simulink model "FEEDBACK_LINEARIZATION"  (R2023b)
settings: Solver=VariableStepAuto  StartTime=0.0  StopTime=70  MaxStep=0.01  RelTol=1e-3
undefined symbols (not defined in the file): A_ego, B_ego, f_r, g, L, N, theta
libraries: sim3dautolib x2, drivingscenarioandsensors x2, mpclib x1, sim3dlib x1
settings Model: Creator=monis  LastModifiedBy=monis

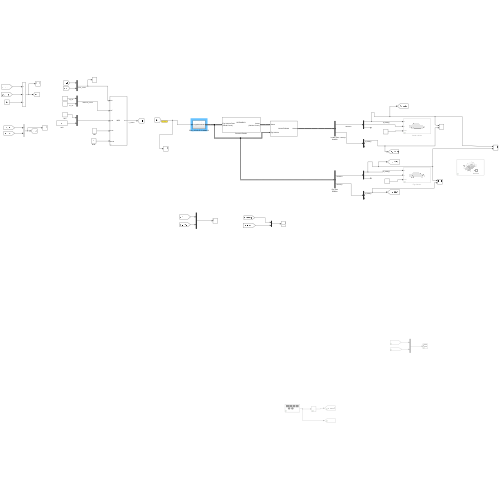
[thumbnail: Simulink's stored preview of the top-level diagram]
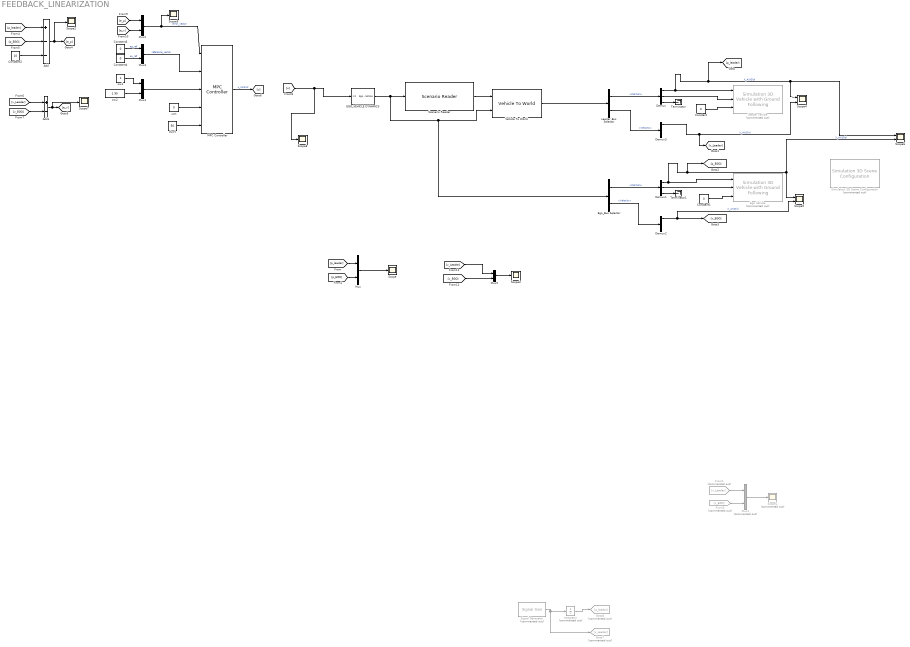
== system FEEDBACK_LINEARIZATION ==
  Add : Sum  Inputs=+--
  Add1 : Sum  Inputs=+-
  Constant{,1,3..4} (4 alike) : Constant  Value=0
  Constant2 : Constant  Value=10
  Demux{,1..3} (4 alike) : Demux  Outputs=3
  EGO_VEHICLE DYNAMICS : Subsystem
  Ego Vehicle : sim3dautolib/Simulation 3D Vehicle with Ground Following  Priority=-1  Commented=on  PassVehMesh=Muscle car  MeshPath=/MathWorksAutomotiveContent/Vehicles/Muscle/Meshes/SK_MuscleCar.SK_MuscleCar  TrackWidth=1.9  WheelBase=3  WheelRadius=0.35  VehColor=Orange  InitialPos=[0, 0, 0]  InitialRot=[0, 0, 0]  ActorName=EgoVehicle  SampleTime=-1  ActorType=SimulinkVehicle  ID=C  aMode=3  ActorTag=EgoVehicle  CoordinateScheme=ISO  VehLightsControl=off  HeadlightColor=[ 1, 1, 1 ]  HighBeamIntensity=100000  LowBeamIntensity=60000  HighBeamConeAngle=70  LowBeamConeAngle=70  LeftHeadlightOrientation=[ 0, 0 ]  RightHeadlightOrientation=[ 0, 0 ]  BrakelightIntensity=500  ReverselightIntensity=500  SignallightIntensity=500  SignallightPeriod=1  SignalPulseWidth=50  TransformOutportEnabled=off
      settings: LibrarySourceBlock=drivingsim3d/Simulation 3D Vehicle with Ground Following
  Ego_Bus Selector : BusSelector  OutputSignals=Position,Velocity
  From1 : From  Commented=on  GotoTag=v_Leader
  From3 : From  Commented=on  GotoTag=v_EGO
  Goto7 : Goto  Commented=on  GotoTag=v_Leader
  Goto8 : Goto  Commented=on  GotoTag=p_leader
  Integrator : Integrator  Commented=on  UpperSaturationLimit=+2500  LowerSaturationLimit=-2500
  Leader vehicle : sim3dautolib/Simulation 3D Vehicle with Ground Following  Priority=-1  Commented=on  PassVehMesh=Muscle car  MeshPath=/MathWorksAutomotiveContent/Vehicles/Muscle/Meshes/SK_MuscleCar.SK_MuscleCar  TrackWidth=1.9  WheelBase=3  WheelRadius=0.35  VehColor=Silver  InitialPos=[0, 0, 0]  InitialRot=[0, 0, 0]  ActorName=LeaderVehicle  SampleTime=-1  ActorType=SimulinkVehicle  ID=C  aMode=3  ActorTag=LeaderVehicle  CoordinateScheme=ISO  VehLightsControl=off  HeadlightColor=[ 1, 1, 1 ]  HighBeamIntensity=100000  LowBeamIntensity=60000  HighBeamConeAngle=70  LowBeamConeAngle=70  LeftHeadlightOrientation=[ 0, 0 ]  RightHeadlightOrientation=[ 0, 0 ]  BrakelightIntensity=500  ReverselightIntensity=500  SignallightIntensity=500  SignallightPeriod=1  SignalPulseWidth=50  TransformOutportEnabled=off
      settings: LibrarySourceBlock=drivingsim3d/Simulation 3D Vehicle with Ground Following
  Leader_Bus Selector : BusSelector  OutputSignals=Actors.Position,Actors.Velocity
  MPC Controller : mpclib/MPC Controller  SCDEnableBlockLinearizationSpecification=on  mpcobj=mpc2  is_multiple=0  enable_value=0  return_u0=off  updateMPCinCallerWorkspace=on  md_inport=off  mv_inport=off  uref_inport=off  return_cost=off  return_mvseq=off  return_qpstatus=off  return_xseq=off  return_state=off  return_ovseq=off  state_inport=off  umin_inport=off  umax_inport=off  ymin_inport=off  ymax_inport=off  cc_inport=off  ywt_inport=on  uwt_inport=on  duwt_inport=on  rhoeps_inport=off  pm_inport=off  MaximumP=10  HorizonChoice=FixedHorizon  n_ts=0.01  n_p=100  n_mv=1  n_md=0  n_ud=0  n_mo=2  n_uo=0  BlockDataType=double  SampleTimeInherited=off  switch_inport=off
  Mux{,2..5} (5 alike) : Mux  Inputs=2
  Mux1 : Mux  Commented=on  Inputs=2
  Scenario Reader : drivingscenarioandsensors/Scenario Reader  ScenarioSource=From file  ScenarioFileName=C:\Users\monis\Downloads\UNINA LEC\FINAL CONTROL SYS PROJECT 2023\SCENARIO1.mat  ScenarioVariableName=scenario  OutputCoordinateSystem=Vehicle coordinates  EgoVehicleSource=Input port  EgoVehicleActorID=1  OrientVehiclesOnRoad=off  OutputEgoVehiclePose=off  OutputEgoVehicleState=off  SampleTime=0.1  LaneBoundaryOutput=None  LaneBoundaryDistance=0:0.5:9.5  LaneBoundaryLocation=Center of lane markings  BusNameSource=Auto  BusName=BusActors  BusNumActorsSource=Scenario  BusNumActors=100  BusName2Source=Auto  BusName2=BusLaneBoundaries  BusNumLaneBoundariesSource=Scenario  BusNumLaneBoundaries=10  BusName3Source=Auto  BusName3=BusEgoActor  BusName4Source=Auto  BusName4=BusEgoState  ShowCoordinateLabels=on  SimulateUsing=Interpreted execution
  Scope{,2..3,7..9} (6 alike) : Scope
  Scope1 : Scope  Commented=on
  Scope4 : Scope  NumInputPorts=2
  Scope5 : Scope  NumInputPorts=2
  Scope6 : Scope  NumInputPorts=2
  Signal Generator : SignalGenerator  Commented=on  WaveForm=random  Units=rad/sec
  Simulation 3D Scene Configuration : sim3dlib/Simulation 3D Scene Configuration  Priority=0  Commented=on  ProjectFormat=Default Scenes  SceneDesc=Straight road  ProjectName=C:\Users\monis\Downloads\_temp_matlab_R2023b_win64\extern\lib\win64\microsoft\toolbox\shared\sim3d_projects\automotive_project_windows\UE\WindowsNoEditor\VehicleSimulation.exe  ScenePath=/Game/Maps/HwStrght  EnableOpenDRIVE=off  vehTagList={'Custom';'EgoVehicle';'LeaderVehicle';'Scene Origin'}  vehTag=EgoVehicle  FreeCameraInitialTranslation=[0, 0, 0]  FreeCameraDefaultInitialTranslation=[-6, 0, 2]  FreeCameraInitialRotation=[0, 0, 0]  FreeCameraDefaultInitialRotation=[0, -15, 0]  OpVisEn=off  Ts=1/60  EnableWindow=on  EnableRemoteAccess=off  EnableWeather=off  SunAltitude=40.0  SunAzimuth=90  clouds=10  wind=1  fog=0  rain=0  EnableGeospatial=off  OriginHeight=200  OriginLatitude=40.744652  OriginLongitude=-73.988864  MapStyle=Aerial  AdditionalAssetIDs=[]  UseAdvancedSunSky=off  SolarTime=11  TimeZone=-5  Day=21  Month=9  Year=2022  UseDaylightSavingTime=on  DSTStartDay=10  DSTStartMonth=3  DSTEndDay=3  DSTEndMonth=11  DSTSwitchHour=2  sensorTag=MainCamera1  sensorId=1  sensorName=MainCamera1  mountLoc=Origin  offsetFlag=off  tmountOffset=[0, 0, 0]  rmountOffset=[0, 0, 0]  HorizontalResolution=1280  VerticalResolution=720  HorizontalFOV=60  mountPoint=[0 0 0]  mountOrientation=[0 0 0]  aMode=3  ID=1  GeoTrigger=Inactive
      settings: LibrarySourceBlock=drivingsim3d/Simulation 3D Scene Configuration
  Terminator : Terminator
  Terminator1 : Terminator
  Vehicle To World : drivingscenarioandsensors/Vehicle To World  BusNameSource=Auto  BusName=BusVehicleToWorldActors  SimulateUsing=Interpreted execution
  duwt : Constant  Value=50
  ow1 : Constant
  ow2 : Constant  Value=1.95
  uwt : Constant  Value=0
  wires:
  Constant/1 -> Leader vehicle/3
  Constant1/1 -> Ego Vehicle/3
  Ego_Bus Selector/1 -> Demux1/1  "<Position>"
  Demux/1 -> [p_leader], Scope4/1, Scope6/1, Leader vehicle/1  "X_AXIS(p)"
  Demux/2 -> Leader vehicle/2
  Demux1/1 -> [p_EGO], Scope5/1, Scope6/2, Ego Vehicle/1  "X_AXIS(p)"
  Demux1/2 -> Ego Vehicle/2
  Ego_Bus Selector/2 -> Demux2/1  "<Velocity>"
  Demux2/1 -> Scope5/2, [v_EGO]  "X_AXIS(v)"
  Demux3/1 -> [v_Leader], Scope4/2  "X_AXIS(v)"
  [p_leader] -> Mux/1
  Mux/1 -> Scope/1
  From3/1 -> Mux1/2
  Mux1/1 -> Scope1/1
  From1/1 -> Mux1/1
  [p_EGO] -> Mux/2
  Demux/3 -> Terminator/1
  Demux1/3 -> Terminator1/1
  [p_leader] -> Add/1
  [p_EGO] -> Add/2
  Constant2/1 -> Add/3
  [v_Leader] -> Add1/1
  [v_EGO] -> Add1/2
  Add/1 -> Scope2/1, [e_p]
  Add1/1 -> Scope7/1, [e_v]
  [e_p] -> Mux2/1
  [e_v] -> Mux2/2
  Mux2/1 -> Scope9/1, MPC Controller/1  "error_vector"
  Constant3/1 -> Mux3/1  "ep_ref"
  Constant4/1 -> Mux3/2  "ev_ref"
  ow1/1 -> Mux4/1
  ow2/1 -> Mux4/2
  Mux3/1 -> MPC Controller/2  "reference_vector"
  Mux4/1 -> MPC Controller/3
  uwt/1 -> MPC Controller/4
  duwt/1 -> MPC Controller/5
  MPC Controller/1 -> [u]  "u_control"
  [u] -> Scope8/1, EGO_VEHICLE DYNAMICS/1(In1)
  Leader_Bus Selector/2 -> Demux3/1  "<Velocity>"
  Leader_Bus Selector/1 -> Demux/1  "<Position>"
  Scenario Reader/1 -> Vehicle To World/1
  Vehicle To World/1 -> Leader_Bus Selector/1
  EGO_VEHICLE DYNAMICS/1(EgoVehiclePose) -> Ego_Bus Selector/1, Vehicle To World/2, Scenario Reader/1
  Signal Generator/1 -> Goto7/1, Integrator/1
  [v_Leader] -> Mux5/1
  [v_EGO] -> Mux5/2
  Mux5/1 -> Scope3/1
  Integrator/1 -> Goto8/1

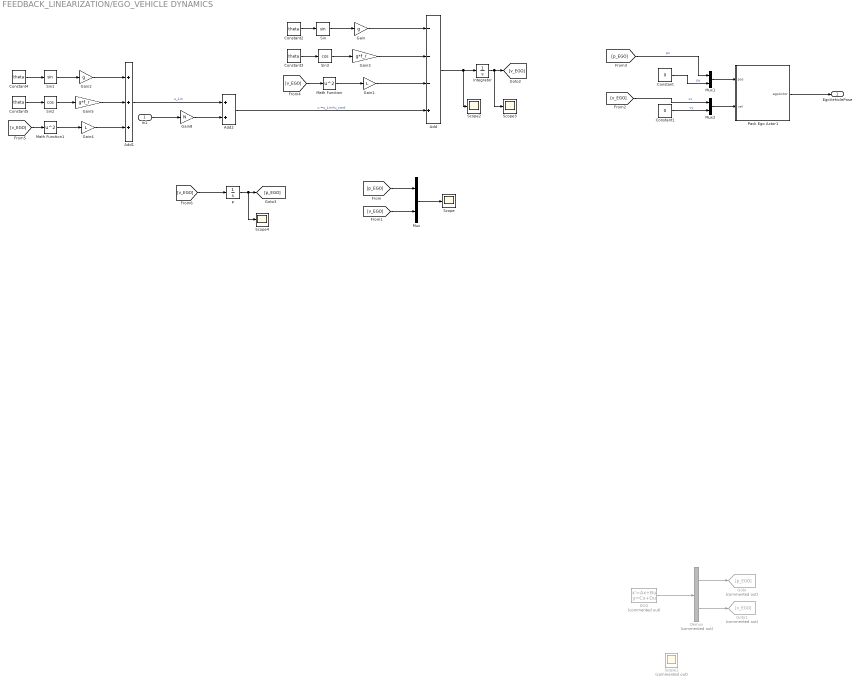
== system FEEDBACK_LINEARIZATION/EGO_VEHICLE DYNAMICS ==
  In1 : Inport
  Add : Sum  Inputs=---+
  Add1 : Sum  Inputs=+++
  Add2 : Sum
  Constant : Constant  Value=0
  Constant1 : Constant  Value=0
  Constant{2..5} (4 alike) : Constant  Value=theta
  Demux : Demux  Commented=on  Outputs=2
  EGO : StateSpace  Commented=on  A=A_ego  B=B_ego  C=eye(2)  D=[0;0]  InitialCondition=[80;20]
  Gain : Gain  Gain=g
  Gain1 : Gain  Gain=L
  Gain2 : Gain  Gain=g
  Gain3 : Gain  Gain=g*f_r
  Gain4 : Gain  Gain=L
  Gain5 : Gain  Gain=g*f_r
  Gain8 : Gain  Gain=N
  Goto : Goto  Commented=on  GotoTag=p_EGO
  Goto1 : Goto  Commented=on  GotoTag=v_EGO
  Integrator : Integrator
  Math Function : Math  Operator=square
  Math Function1 : Math  Operator=square
  Mux : Mux  Inputs=2
  Mux1 : Mux  Inputs=2
  Mux2 : Mux  Inputs=2
  Pack Ego Actor1 : MATLAB Function  TreatAsAtomicUnit=on
  Scope{,2..4} (4 alike) : Scope
  Scope1 : Scope  Commented=on
  Sin : Trigonometry
  Sin1 : Trigonometry
  Sin2 : Trigonometry  Operator=cos
  Sin3 : Trigonometry  Operator=cos
  p : Integrator  InitialCondition=15
  EgoVehiclePose : Outport
  wires:
  Demux/2 -> Goto1/1
  Mux/1 -> Scope/1
  Demux/1 -> Goto/1
  EGO/1 -> Demux/1
  Mux1/1 -> Pack Ego Actor1/1(pos)
  Mux2/1 -> Pack Ego Actor1/2(vel)
  Constant/1 -> Mux1/2  "py"
  [p_EGO] -> Mux1/1  "px"
  Constant1/1 -> Mux2/2  "vy"
  [v_EGO] -> Mux2/1  "vx"
  Pack Ego Actor1/1(egoActor) -> EgoVehiclePose/1
  Constant2/1 -> Sin/1
  Sin/1 -> Gain/1
  Constant3/1 -> Sin3/1
  Sin3/1 -> Gain3/1
  Gain3/1 -> Add/2
  Gain/1 -> Add/1
  Gain1/1 -> Add/3
  Math Function/1 -> Gain1/1
  [v_EGO] -> Math Function/1
  Constant4/1 -> Sin1/1
  Sin1/1 -> Gain2/1
  Gain2/1 -> Add1/1
  Gain5/1 -> Add1/2
  Gain4/1 -> Add1/3
  Sin2/1 -> Gain5/1
  Constant5/1 -> Sin2/1
  Math Function1/1 -> Gain4/1
  [v_EGO] -> Math Function1/1
  Add1/1 -> Add2/1  "u_Lin"
  In1/1 -> Gain8/1
  Add/1 -> Scope2/1, Integrator/1
  Integrator/1 -> Scope3/1, [v_EGO]
  Add2/1 -> Add/4  "u =u_Lin+u_cont"
  [v_EGO] -> p/1
  p/1 -> Scope4/1, [p_EGO]
  [p_EGO] -> Mux/1
  [v_EGO] -> Mux/2
  Gain8/1 -> Add2/2

== matlab function FEEDBACK_LINEARIZATION/EGO_VEHICLE DYNAMICS/Pack Ego Actor1 ==
  data: pos input; egoActor output Bus: BusActors1Actors size=1; vel input
function egoActor = packEgo(pos,vel)
% Pack ego information into a single ego actor bus
%
% Imoprtant note:
% Output is a bus of type BusActorsActors. This is the same bus used by the
% Scenario Reader to output an individual actor. If you change the
% output bus name of Scenario Reader, change the output bus name here
% as well by clicking on 'Edit Data' in the menu above.

egoActor = struct(...
    'ActorID',1,...
    'Position', [pos(1) pos(2) 0], ...
    'Velocity', [vel(1) vel(2) 0], ...
    'Roll', 0, ...
    'Pitch', 0, ...
    'Yaw', 0, ...
    'AngularVelocity', [0 0 0]);
